simulink model "Subsystem"  (R2020a)
settings: Solver=VariableStepAuto  StartTime=0.0  StopTime=10.0  RelTol=1e-3
settings Model: Creator=Riyansh  LastModifiedBy=Riyansh
settings DataIOCC: SaveOutput=off  SaveTime=off

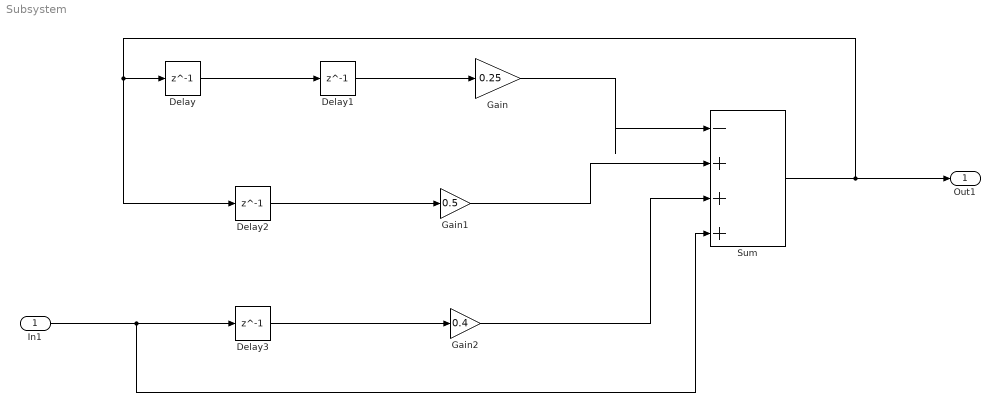
== system Subsystem ==
  In1 : Inport  OutDataTypeStr=double  PortDimensions=1  SampleTime=[0,1]
  Delay{,1..3} (4 alike) : Delay  DelayLength=1
  Gain : Gain  Gain=0.25
  Gain1 : Gain  Gain=0.5
  Gain2 : Gain  Gain=0.4
  Sum : Sum  Inputs=|-+++
  Out1 : Outport  OutDataTypeStr=double  PortDimensions=1  SampleTime=[0,1]
  wires:
  Delay3/1 -> Gain2/1
  In1/1 -> Delay3/1, Sum/4
  Delay/1 -> Delay1/1
  Gain2/1 -> Sum/3
  Gain1/1 -> Sum/2
  Delay1/1 -> Gain/1
  Delay2/1 -> Gain1/1
  Gain/1 -> Sum/1
  Sum/1 -> Delay2/1, Delay/1, Out1/1
